simulink model "adaptive_observer_for_sin_signal_original"  (R2021b)
settings: Solver=ode4  StartTime=0.0  StopTime=simulationTime  FixedStep=0.0001  RelTol=1e-3
model workspace: external: MATLAB File D:\practice\sci\variables2n1.m (data not in the file)
values from neighbouring files (symbols this model uses):
  A = zeros(2*dimension+1 , 2*dimension+1)    [LCAD.m]
  alpha = [1,3]    [variables2n1.m]
  amp = [1;1]    [variables2n1.m]
  amp_M = [1;1]    [variables2n1.m]
  amp_M1 = 0.2    [variables2n1.m]
  bias = [0;0]    [variables2n1.m]
  bias_M = [0;0]    [variables2n1.m]
  bias_M1 = 0    [variables2n1.m]
  bigGammaZ0 = zeros(2*dimension+1, dimension)    [variables2n1.m]
  C = zeros(1, 2*dimension+1)    [LCAD.m]
  delta = C*A    [LCAD.m]    (also in stats.m = 0.05)
  dimension = 2    [variables2n1.m]
  freq = [2;3]    [variables2n1.m]
  freq_M = [1.8;3.2]    [variables2n1.m]
  freq_M1 = 20    [variables2n1.m]
  freqSwitcher = [80,150]    [variables2n1.m]
  gamma_my = 0.01    [starter3.m]
  h_my = 0.3    [starter3.m]
  initialTheta = [initialOmega(1)^2-alpha(1);     initialOmega(2)^2-alpha(2)]    [variables2n1.m]
  initialZ = [sin(phase(1)); r^2*cos(phase(1))/initialOmega(1);     sin(phase(2)); r^2*cos(phase(2))/initialOmega(2); sum(bias)]    [variables2n1.m]
  k_my = 100    [starter3.m]
  L = real((place(A',C',eigenvalues))')    [LCAD.m]
  mu = 25    [graphs.m]    (also in plot_pres4.m = 2.5; variables2n1.m = 2.5)
  noiseOrSin = 0    [variables2n1.m]
  noiseOrSwitch = 0    [variables2n1.m]
  omega1 = ones(1, length(time))*2    [graphs.m]    (also in starter3.m = 2)
  omega2 = ones(1, length(time))*3    [graphs.m]    (also in starter3.m = 3)
  omega_max = 10    [starter3.m]
  omega_min = 1    [starter3.m]
  omegaLimiter = sqrt(dimension)*maxOmega    [variables2n1.m]
  phase = [0;0]    [variables2n1.m]
  phase_M = [0;0]    [variables2n1.m]
  phase_M1 = 0    [variables2n1.m]
  r = 1.2    [variables2n1.m]
  sample_M1 = 10    [variables2n1.m]
  tau_my = 0.3    [starter3.m]
  theta0_my = [-2; 1]    [starter3.m]
  theta_real = [-c1-c2; c1*c2]    [starter3.m]
  turn_mods_on = 1    [variables2n1.m]
  zMax = 5    [variables2n1.m]
undefined symbols (not defined in the file or in its folder): G, isComplex, L1
libraries: simulink x1
(part 3 of 3)

== matlab function adaptive_observer_for_sin_signal_original/Estimator mu=10/Г(z) ==
  settings: sampleTime=0.1
  data: z input size=[2*dimension+1 1]; bigGammaZ output size=[2*dimension+1 dimension]; dimension parameter size=1; bigGammaZ0 parameter size=[2*dimension+1 dimension]
function bigGammaZ = gms1(z, dimension, bigGammaZ0)

bigGammaZ = bigGammaZ0;
for i = 1:dimension
    bigGammaZ(2*i - 1,i) = z(2*i);
end

== matlab function adaptive_observer_for_sin_signal_original/Estimator mu=2.5/Frequencies estimator/Fc/max S1 ==
  settings: sampleTime=0.1
  data: bigOmega input size=[dimension 1]; z input size=[2*dimension+1 1]; r parameter size=1; delta parameter size=[1 2*dimension+1]; PHI input size=[dimension 1]; maxS output size=1; gammaZ input size=[dimension 1]; t input size=1; dimension parameter size=1; mu input size=1
function maxS = SCounter(bigOmega, z, r, delta, PHI, gammaZ, t, dimension,...
mu)

    tempSum = 0;

    z2 = z(2:2:end);

    frequency = zeros(dimension,1);
    parfor i = 1:dimension
        frequency(i) = sqrt(abs(bigOmega(i))); 
    end

    
    if(t > 60 && t < 140)
        disturbanceDot = 1;
    else 
        disturbanceDot = 0;
    end

    parfor i = 1:dimension
        tempSum = tempSum + frequency(i)^2 * z2(i) + disturbanceDot; %1 
    end

    gammaZ = gammaZ';


    maxS = norm(r^2 * mu * gammaZ * tempSum - r^2 * mu * gammaZ ... 
       * (gammaZ * PHI + delta * z));


    maxS = maxS*1.1;

end

== matlab function adaptive_observer_for_sin_signal_original/MATLAB Function1 ==
  data: bigOmega input; omega_hat output
function omega_hat = fcn(bigOmega)

omega_hat = sqrt(abs(bigOmega));

== matlab function adaptive_observer_for_sin_signal_original/FT Ved/Gradient1/MATLAB Function ==
  data: theta_hat input size=[2,1]; W input; theta_ft output size=[2, 1]; theta0_my parameter
function theta_ft = fcn(theta_hat, W, theta0_my)

%theta_ft = zeros(size(theta_hat));
if W > 0.8
    W = 0.8;
end
theta_ft = (theta_hat - theta0_my*W)./(1-W);

== matlab function adaptive_observer_for_sin_signal_original/FT Ved/MATLAB Function2 ==
  data: theta_hat input; omega_hat output; h_my parameter; Q output; omega_max parameter; omega_min parameter
function [omega_hat, Q]  = fcn(theta_hat, h_my, omega_max, omega_min)

% theta1 = theta_hat(1);
% theta2 = theta_hat(2);
% 
% omega1_hat = real(1/h*acos(1/2*complex(theta1 + sqrt(complex(theta1^2 - theta2)))))
% omega2_hat = real(1/h*acos(1/2*complex(theta1 - sqrt(complex(theta1^2 - theta2)))))
% 
% omega_hat = [omega1_hat; omega2_hat]

c_hat = zeros(2, 1);
x = roots([1 theta_hat(1) theta_hat(2)]);
c_hat = [x(1); x(2)];
Q = real(c_hat);
%c_hat = max([-1; -1], min([1; 1], real(c_hat)));
omega_hat = min(real(1/h_my*acos(complex(c_hat))), omega_max*[1; 1]);

== matlab function adaptive_observer_for_sin_signal_original/FT Ved/Regression model/MATLAB Function ==
  data: y input; y1 input; psi output; y2 input; y3 input; y4 input; theta output; phi output; omega1 parameter; omega2 parameter; h_my parameter
function [psi,theta, phi] = fcn(y, y1, y2, y3, y4, omega1, omega2, h_my)

c1 = cos(omega1*h_my);
c2 = cos(omega2*h_my);

% psi = y + 2*y2 + y4;
% theta = [c1+c2; 4*c1*c2];
% phi = [2*y1 + 2*y3; -y2];

psi = -(y + 2*y2 + y4);
theta = [-c1-c2; c1*c2];
phi = [2*(y1 + y3); 4*y2];

== matlab function adaptive_observer_for_sin_signal_original/Proposed Estimator1/Frequencies estimator/Fc/max S ==
  settings: sampleTime=0.1
  data: bigOmega input size=[dimension 1]; z input size=[2*dimension+1 1]; r parameter size=1; delta parameter size=[1 2*dimension+1]; PHI input size=[dimension 1]; maxS output size=1; gammaZ input size=[dimension 1]; t input size=1; dimension parameter size=1; mu input size=1
function maxS = SCounter(bigOmega, z, r, delta, PHI, gammaZ, t, dimension,...
mu)

    tempSum = 0;

    z2 = z(2:2:end);

    frequency = zeros(dimension,1);
    parfor i = 1:dimension
        frequency(i) = sqrt(abs(bigOmega(i))); 
    end

    
    if(t > 60 && t < 140)
        disturbanceDot = 1;
    else 
        disturbanceDot = 0;
    end

    parfor i = 1:dimension
        tempSum = tempSum + frequency(i)^2 * z2(i) + disturbanceDot; %1 
    end

    gammaZ = gammaZ';


    maxS = norm(r^2 * mu * gammaZ * tempSum - r^2 * mu * gammaZ ... 
       * (gammaZ * PHI + delta * z));


    maxS = maxS*1.1;

end

== matlab function adaptive_observer_for_sin_signal_original/Proposed Estimator1/Frequencies estimator/Fc/||Ω|| ==
  data: bigOmega input size=[dimension 1]; normOmega output size=1
function normOmega = norma(bigOmega)

normOmega = norm(bigOmega);

== matlab function adaptive_observer_for_sin_signal_original/Proposed Estimator/z'/S(z)/valType filter ==
  data: multiplied input; filtered output
function filtered = fcn(multiplied)

if class(multiplied) == 'double'
    filtered = multiplied;
elseif class(multiplied) == 'complex'
    filtered = abs(multiplied);
end

== matlab function adaptive_observer_for_sin_signal_original/Proposed Estimator1/Frequencies estimator/Fc/Ψ ==
  data: isGreater input; Psi output
function Psi = PSI(isGreater)

if isGreater
    Psi = 1;
else 
    Psi = 0;
end

== matlab function adaptive_observer_for_sin_signal_original/Proposed Estimator1/Subsystem1/MATLAB Function ==
  data: zPrime input; z output; t input; initialZ parameter
function z = fcn(zPrime, t, initialZ)

if (t == 0)
    cont = [0, initialZ];
    
end

== matlab function adaptive_observer_for_sin_signal_original/Proposed Estimator1/z'/S(z)/MATLAB Function ==
  data: con1 input; res output; con2 input
function res = fcn(con1, con2)

if (con1 == true) && (con2 == true)
    res = 1;
else
    res = 0;
end

== matlab function adaptive_observer_for_sin_signal_original/Proposed Estimator1/z'/S(z)/normalize ==
  data: z input size=[2*dimension+1 1]; normZ output size=1
function normZ = norma(z)

normZ = norm(z);

== matlab function adaptive_observer_for_sin_signal_original/MATLAB Function4 ==
  data: bigOmega input; omega_hat output
function omega_hat = fcn(bigOmega)

omega_hat = sqrt(abs(bigOmega));

== matlab function adaptive_observer_for_sin_signal_original/Proposed Estimator1/Г(z) ==
  settings: sampleTime=0.1
  data: z input size=[2*dimension+1 1]; bigGammaZ output size=[2*dimension+1 dimension]; dimension parameter size=1; bigGammaZ0 parameter size=[2*dimension+1 dimension]
function bigGammaZ = gms1(z, dimension, bigGammaZ0)

bigGammaZ = bigGammaZ0;
for i = 1:dimension
    bigGammaZ(2*i - 1,i) = z(2*i);
end

== matlab function adaptive_observer_for_sin_signal_original/Proposed Estimator/z'/S(z)/MATLAB Function ==
  data: con1 input; res output; con2 input
function res = fcn(con1, con2)

if (con1 == true) && (con2 == true)
    res = 1;
else
    res = 0;
end

== matlab function adaptive_observer_for_sin_signal_original/Proposed Estimator/Frequencies estimator/Fc/||Ω|| ==
  data: bigOmega input size=[dimension 1]; normOmega output size=1
function normOmega = norma(bigOmega)

normOmega = norm(bigOmega);

== matlab function adaptive_observer_for_sin_signal_original/Proposed Estimator/Frequencies estimator/Fc/Ψ ==
  data: isGreater input; Psi output
function Psi = PSI(isGreater)

if isGreater
    Psi = 1;
else 
    Psi = 0;
end

== matlab function adaptive_observer_for_sin_signal_original/Proposed Estimator/Subsystem1/MATLAB Function ==
  data: zPrime input; z output; t input; initialZ parameter
function z = fcn(zPrime, t, initialZ)

if (t == 0)
    cont = [0, initialZ];
    
end

== matlab function adaptive_observer_for_sin_signal_original/Proposed Estimator/Г(z) ==
  settings: sampleTime=0.1
  data: z input size=[2*dimension+1 1]; bigGammaZ output size=[2*dimension+1 dimension]; dimension parameter size=1; bigGammaZ0 parameter size=[2*dimension+1 dimension]
function bigGammaZ = gms1(z, dimension, bigGammaZ0)

bigGammaZ = bigGammaZ0;
for i = 1:dimension
    bigGammaZ(2*i - 1,i) = z(2*i);
end

== matlab function adaptive_observer_for_sin_signal_original/Original Signal/MATLAB Function ==
  data: z input; t input; zSup output; zPrev input
function zSup = fcn(z, t, zPrev)



if (t == 0)
    zPrev = norm(z);
end

zSup = max(norm(z),zPrev);

== matlab function adaptive_observer_for_sin_signal_original/Proposed Estimator/z'/S(z)/normalize ==
  data: z input size=[2*dimension+1 1]; normZ output size=1
function normZ = norma(z)

normZ = norm(z);
